simulink model "RobotArm_PID"  (R2020a)
settings: Solver=VariableStepAuto  StartTime=0.0  StopTime=20  RelTol=1e-3
undefined symbols (not defined in the file or in its folder): DiscIntNeverNeededParam
libraries: simulink x2
settings Model: Creator=nikhil  LastModifiedBy=nikhil

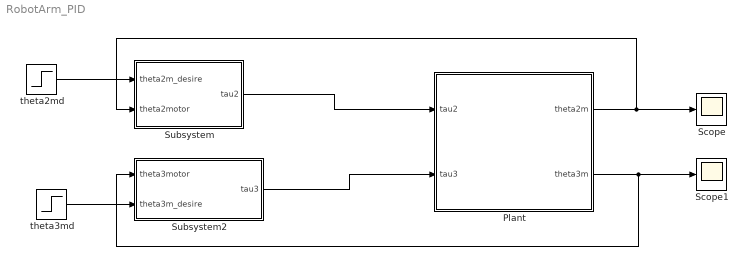
== system RobotArm_PID ==
  Plant : Subsystem
  Scope : Scope
  Scope1 : Scope
  Subsystem : Subsystem
  Subsystem2 : Subsystem
  theta2md : Step  After=0.5  SampleTime=0
  theta3md : Step  After=0.5  SampleTime=0
  wires:
  theta2md/1 -> Subsystem/1(theta2m_desire)
  theta3md/1 -> Subsystem2/2(theta3m_desire)
  Subsystem/1(tau2) -> Plant/1(tau2)
  Subsystem2/1(tau3) -> Plant/2(tau3)
  Plant/2(theta3m) -> Subsystem2/1(theta3motor), Scope1/1
  Plant/1(theta2m) -> Subsystem/2(theta2motor), Scope/1

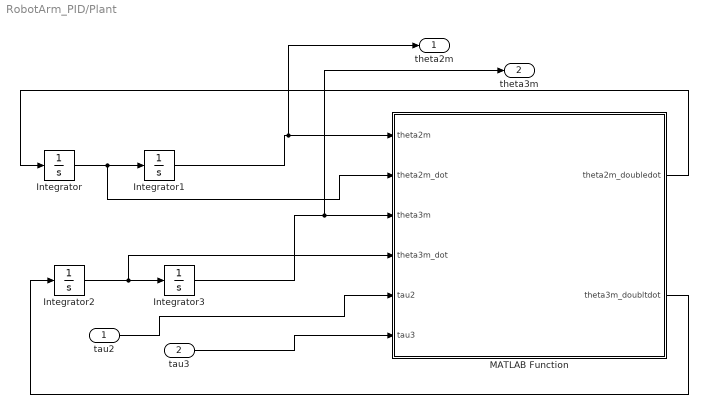
== system RobotArm_PID/Plant ==
  tau2 : Inport
  tau3 : Inport  Port=2
  Integrator{,1..3} (4 alike) : Integrator
  MATLAB Function : MATLAB Function  TreatAsAtomicUnit=on
  theta2m : Outport
  theta3m : Outport  Port=2
  wires:
  Integrator1/1 -> theta2m/1, MATLAB Function/1(theta2m)
  MATLAB Function/2(theta3m_doubltdot) -> Integrator2/1
  MATLAB Function/1(theta2m_doubledot) -> Integrator/1
  Integrator3/1 -> theta3m/1, MATLAB Function/3(theta3m)
  Integrator2/1 -> MATLAB Function/4(theta3m_dot), Integrator3/1
  tau3/1 -> MATLAB Function/6(tau3)
  Integrator/1 -> MATLAB Function/2(theta2m_dot), Integrator1/1
  tau2/1 -> MATLAB Function/5(tau2)

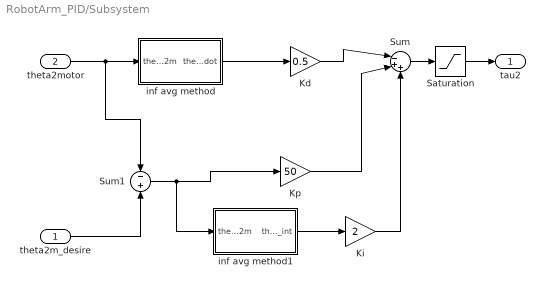
== system RobotArm_PID/Subsystem ==
  theta2m_desire : Inport
  theta2motor : Inport  Port=2
  Kd : Gain  Gain=0.5
  Ki : Gain  Gain=2
  Kp : Gain  Gain=50
  Saturation : Saturate  UpperLimit=5  LowerLimit=-5
  Sum : Sum  Inputs=|-++
  Sum1 : Sum  Inputs=-|+
  inf avg method : Subsystem
  inf avg method1 : Subsystem
  tau2 : Outport
  wires:
  Sum/1 -> Saturation/1
  theta2motor/1 -> Sum1/1, inf avg method/1(theta2m)
  Sum1/1 -> inf avg method1/1(theta2m), Kp/1
  Kp/1 -> Sum/2
  Kd/1 -> Sum/1
  theta2m_desire/1 -> Sum1/2
  inf avg method/1(theta2m_dot) -> Kd/1
  inf avg method1/1(theta2m_int) -> Ki/1
  Ki/1 -> Sum/3
  Saturation/1 -> tau2/1

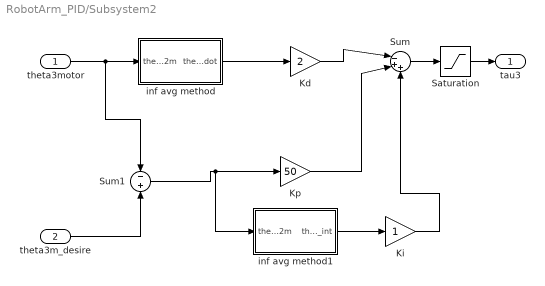
== system RobotArm_PID/Subsystem2 ==
  theta3motor : Inport
  theta3m_desire : Inport  Port=2
  Kd : Gain  Gain=2
  Ki : Gain
  Kp : Gain  Gain=50
  Saturation : Saturate  UpperLimit=5  LowerLimit=-5
  Sum : Sum  Inputs=|-++
  Sum1 : Sum  Inputs=-|+
  inf avg method : Subsystem
  inf avg method1 : Subsystem
  tau3 : Outport
  wires:
  Sum/1 -> Saturation/1
  theta3motor/1 -> Sum1/1, inf avg method/1(theta2m)
  Kp/1 -> Sum/2
  Kd/1 -> Sum/1
  theta3m_desire/1 -> Sum1/2
  inf avg method/1(theta2m_dot) -> Kd/1
  Ki/1 -> Sum/3
  Sum1/1 -> inf avg method1/1(theta2m), Kp/1
  inf avg method1/1(theta2m_int) -> Ki/1
  Saturation/1 -> tau3/1

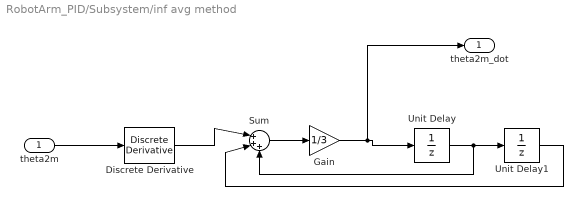
== system RobotArm_PID/Subsystem/inf avg method ==
  theta2m : Inport
  Discrete Derivative : simulink/Discrete/Discrete Derivative  gainval=1.0  ICPrevScaledInput=0.001  OutMin=[]  OutMax=[]  OutDataType=fixdt(1, 16)  OutScaling=2^-10  DoSatur=off
  Gain : Gain  Gain=1/3
  Sum : Sum  Inputs=|+++
  Unit Delay : UnitDelay  SampleTime=-1  HasFrameUpgradeWarning=on
  Unit Delay1 : UnitDelay  SampleTime=-1  HasFrameUpgradeWarning=on
  theta2m_dot : Outport
  wires:
  Gain/1 -> theta2m_dot/1, Unit Delay/1
  Unit Delay/1 -> Sum/3, Unit Delay1/1
  Unit Delay1/1 -> Sum/2
  Discrete Derivative/1 -> Sum/1
  theta2m/1 -> Discrete Derivative/1
  Sum/1 -> Gain/1

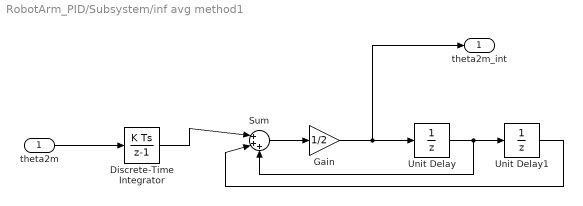
== system RobotArm_PID/Subsystem/inf avg method1 ==
  theta2m : Inport
  Discrete-Time Integrator : DiscreteIntegrator  SampleTime=-1  ICPrevOutput=DiscIntNeverNeededParam  ICPrevScaledInput=DiscIntNeverNeededParam
  Gain : Gain  Gain=1/2
  Sum : Sum  Inputs=|+++
  Unit Delay : UnitDelay  SampleTime=-1  HasFrameUpgradeWarning=on
  Unit Delay1 : UnitDelay  SampleTime=-1  HasFrameUpgradeWarning=on
  theta2m_int : Outport
  wires:
  Gain/1 -> theta2m_int/1, Unit Delay/1
  Unit Delay/1 -> Sum/3, Unit Delay1/1
  Unit Delay1/1 -> Sum/2
  Discrete-Time Integrator/1 -> Sum/1
  theta2m/1 -> Discrete-Time Integrator/1
  Sum/1 -> Gain/1

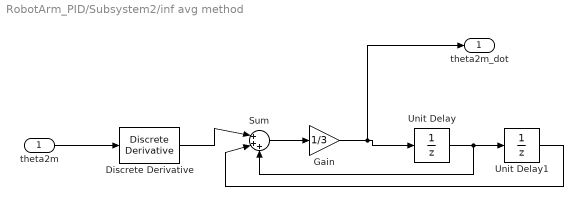
== system RobotArm_PID/Subsystem2/inf avg method ==
  theta2m : Inport
  Discrete Derivative : simulink/Discrete/Discrete Derivative  gainval=1.0  ICPrevScaledInput=0.001  OutMin=[]  OutMax=[]  OutDataType=fixdt(1, 16)  OutScaling=2^-10  DoSatur=off
  Gain : Gain  Gain=1/3
  Sum : Sum  Inputs=|+++
  Unit Delay : UnitDelay  SampleTime=-1  HasFrameUpgradeWarning=on
  Unit Delay1 : UnitDelay  SampleTime=-1  HasFrameUpgradeWarning=on
  theta2m_dot : Outport
  wires:
  Gain/1 -> theta2m_dot/1, Unit Delay/1
  Unit Delay/1 -> Sum/3, Unit Delay1/1
  Unit Delay1/1 -> Sum/2
  Discrete Derivative/1 -> Sum/1
  theta2m/1 -> Discrete Derivative/1
  Sum/1 -> Gain/1

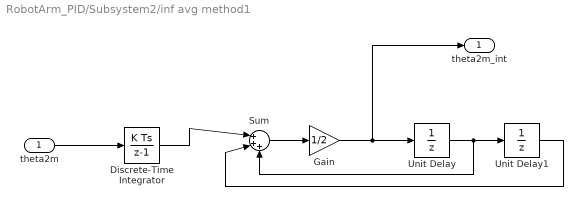
== system RobotArm_PID/Subsystem2/inf avg method1 ==
  theta2m : Inport
  Discrete-Time Integrator : DiscreteIntegrator  SampleTime=-1  ICPrevOutput=DiscIntNeverNeededParam  ICPrevScaledInput=DiscIntNeverNeededParam
  Gain : Gain  Gain=1/2
  Sum : Sum  Inputs=|+++
  Unit Delay : UnitDelay  SampleTime=-1  HasFrameUpgradeWarning=on
  Unit Delay1 : UnitDelay  SampleTime=-1  HasFrameUpgradeWarning=on
  theta2m_int : Outport
  wires:
  Gain/1 -> theta2m_int/1, Unit Delay/1
  Unit Delay/1 -> Sum/3, Unit Delay1/1
  Unit Delay1/1 -> Sum/2
  Discrete-Time Integrator/1 -> Sum/1
  theta2m/1 -> Discrete-Time Integrator/1
  Sum/1 -> Gain/1

== matlab function RobotArm_PID/Plant/MATLAB Function ==
  data: theta2m input; theta2m_doubledot output; theta2m_dot input; theta3m input; theta3m_dot input; tau2 input; tau3 input; theta3m_doubltdot output
function [theta2m_doubledot, theta3m_doubltdot]  = fcn(theta2m, theta2m_dot, theta3m, theta3m_dot,tau2, tau3)
p = [0.03;0.0128;0.0076;0.0753;0.0298];
p1=p(1);
p2=p(2);
p3=p(3);
p4=p(4);
p5=p(5);
g=9.81;
Fic = [-0.04*theta2m_dot; -0.037*theta3m_dot];
tau = [tau2;tau3];
D = [p1 -p3*sin(theta3m - theta2m); -p3*sin(theta3m-theta2m) p2];
C = [0 -p3*cos(theta3m - theta2m)*theta3m_dot;
    p3*cos(theta3m-theta2m)*theta2m_dot 0];
G = [-p4*g*sin(theta2m); -p5*g*cos(theta3m)];
out = inv(D)*tau -inv(D)*C*[theta2m_dot;theta3m_dot] - inv(D)*G + inv(D)*Fic;
theta2m_doubledot = out(1);
theta3m_doubltdot = out(2);
end
